simulink model "nonlinsim"  (R2015a)
settings: Solver=ode45  StartTime=0.0  StopTime=30.0  RelTol=1e-3
values from neighbouring files (symbols this model uses):
  s = tf('s')    [ekstranul.m]
undefined symbols (not defined in the file or in its folder): Grx, rrx
libraries: cstblocks x7, simulink x1
settings Model: Creator=morten  LastModifiedBy=morten

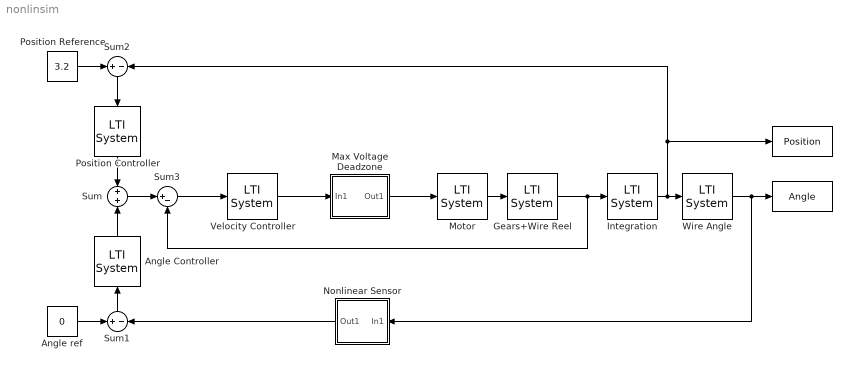
== system nonlinsim ==
  "  " : ToWorkspace  VariableName=Angle  SaveFormat=Timeseries  SampleTime=-1
  "   " : ToWorkspace  VariableName=Position  SaveFormat=Timeseries  SampleTime=-1
  Angle Controller : cstblocks/LTI System  sys=Ctheta  IC=[]
  Angle ref : Constant  Value=0
  Gears+Wire Reel : cstblocks/LTI System  sys=Grx*rrx  IC=[]
  Integration : cstblocks/LTI System  sys=1/s  IC=[]
  Max Voltage Deadzone : Subsystem
  Motor : cstblocks/LTI System  sys=Mx  IC=[]
  Nonlinear Sensor : Subsystem
  Position Controller : cstblocks/LTI System  sys=Cx  IC=[]
  Position Reference : Constant  Value=3.2
  Sum : Sum  Inputs=+|+
  Sum1 : Sum  Inputs=+|-
  Sum2 : Sum  Inputs=+|-
  Sum3 : Sum  Inputs=|+-
  Velocity Controller : cstblocks/LTI System  sys=CV  IC=[]
  Wire Angle : cstblocks/LTI System  sys=W  IC=[]
  wires:
  Motor/1 -> Gears+Wire Reel/1
  Wire Angle/1 -> "  "/1, Nonlinear Sensor/1(In1)
  Velocity Controller/1 -> Max Voltage Deadzone/1(In1)
  Angle ref/1 -> Sum1/1
  Angle Controller/1 -> Sum/2
  Position Controller/1 -> Sum/1
  Sum1/1 -> Angle Controller/1
  Sum2/1 -> Position Controller/1
  Position Reference/1 -> Sum2/1
  Max Voltage Deadzone/1(Out1) -> Motor/1
  Integration/1 -> Sum2/2, "   "/1, Wire Angle/1
  Gears+Wire Reel/1 -> Sum3/2, Integration/1
  Nonlinear Sensor/1(Out1) -> Sum1/2
  Sum/1 -> Sum3/1
  Sum3/1 -> Velocity Controller/1

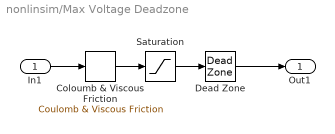
== system nonlinsim/Max Voltage Deadzone ==
  In1 : Inport
  Coloumb & Viscous Friction : simulink/Discontinuities/Coulomb & Viscous Friction  offset=[4.2]  gain=1
  Dead Zone : DeadZone  LowerValue=-4.2  UpperValue=4.2  SaturateOnIntegerOverflow=on
  Saturation : Saturate  UpperLimit=12.5  LowerLimit=-12.5
  Out1 : Outport
  wires:
  Dead Zone/1 -> Out1/1
  Saturation/1 -> Dead Zone/1
  In1/1 -> Coloumb & Viscous Friction/1
  Coloumb & Viscous Friction/1 -> Saturation/1

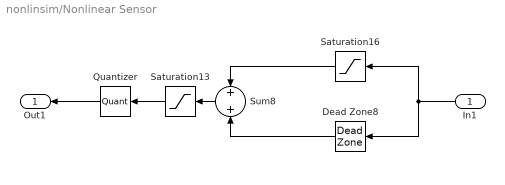
== system nonlinsim/Nonlinear Sensor ==
  In1 : Inport
  Dead Zone8 : DeadZone  LowerValue=-0.3387  UpperValue=0.3227  SaturateOnIntegerOverflow=on
  Quantizer : Quantizer  QuantizationInterval=0.001
  Saturation13 : Saturate  UpperLimit=0.664  LowerLimit=-0.68
  Saturation16 : Saturate  UpperLimit=.1627  LowerLimit=-0.1787
  Sum8 : Sum  Inputs=+|+
  Out1 : Outport
  wires:
  Dead Zone8/1 -> Sum8/2
  Saturation16/1 -> Sum8/1
  Sum8/1 -> Saturation13/1
  In1/1 -> Dead Zone8/1, Saturation16/1
  Saturation13/1 -> Quantizer/1
  Quantizer/1 -> Out1/1
